simulink model "compressor"  (R2014a)
settings: Solver=ode45  StartTime=0.0  StopTime=100  RelTol=1e-4
libraries: simulink x2
settings Model: Creator=Max  LastModifiedBy=Max

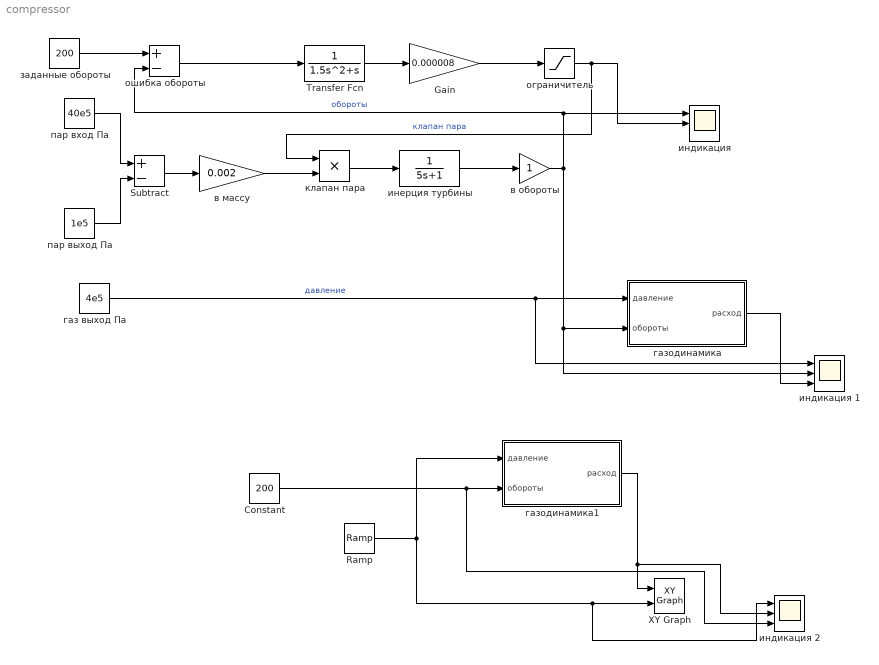
== system compressor ==
  Constant : Constant  Value=200
  Gain : Gain  Gain=0.000008
  Ramp : simulink/Sources/Ramp  slope=1  start=0  X0=1
  Subtract : Sum  Inputs=+-
  Transfer Fcn : TransferFcn  Denominator=[1.5 1 0]
  XY Graph : simulink/Sinks/XY Graph  xmin=-1500  xmax=1500  ymin=-50  ymax=50  st=-1
  в массу : Gain  Gain=0.002
  в обороты : Gain
  газ выход Па : Constant  Value=4e5
  газодинамика : Subsystem  TreatAsAtomicUnit=on
  газодинамика1 : Subsystem  TreatAsAtomicUnit=on
  заданные обороты : Constant  Value=200
  "индикация " : Scope  NumInputPorts=3
      settings: ShowLegends=on  YMin=0~-5~-5  YMax=4250~5~5
  индикация 1 : Scope  NumInputPorts=3
      settings: ShowLegends=on  YMin=-5~-5~-5  YMax=5~5~5
  индикация 2 : Scope  NumInputPorts=3
      settings: ShowLegends=on  YMin=-5~-5~-5  YMax=5~5~5  SaveName=ScopeData2
  инерция турбины : TransferFcn  Denominator=[5 1]
  клапан пара : Product
  ограничитель : Saturate  UpperLimit=1  LowerLimit=0
  ошибка обороты : Sum  Inputs=+-
  пар вход Па : Constant  Value=40e5
  пар выход Па : Constant  Value=1e5
  wires:
  пар выход Па/1 -> Subtract/2
  пар вход Па/1 -> Subtract/1
  Subtract/1 -> в массу/1
  в массу/1 -> клапан пара/2
  клапан пара/1 -> инерция турбины/1
  инерция турбины/1 -> в обороты/1
  заданные обороты/1 -> ошибка обороты/1
  в обороты/1 -> газодинамика/2(обороты), индикация 1/2, ошибка обороты/2, "индикация "/1  "обороты"
  ограничитель/1 -> клапан пара/1, "индикация "/2  "клапан пара"
  газ выход Па/1 -> газодинамика/1(давление), индикация 1/1  "давление"
  газодинамика/1(расход) -> индикация 1/3
  газодинамика1/1(расход) -> индикация 2/2, XY Graph/1
  Constant/1 -> индикация 2/3, газодинамика1/2(обороты)
  Ramp/1 -> индикация 2/1, XY Graph/2, газодинамика1/1(давление)
  Transfer Fcn/1 -> Gain/1
  ошибка обороты/1 -> Transfer Fcn/1
  Gain/1 -> ограничитель/1

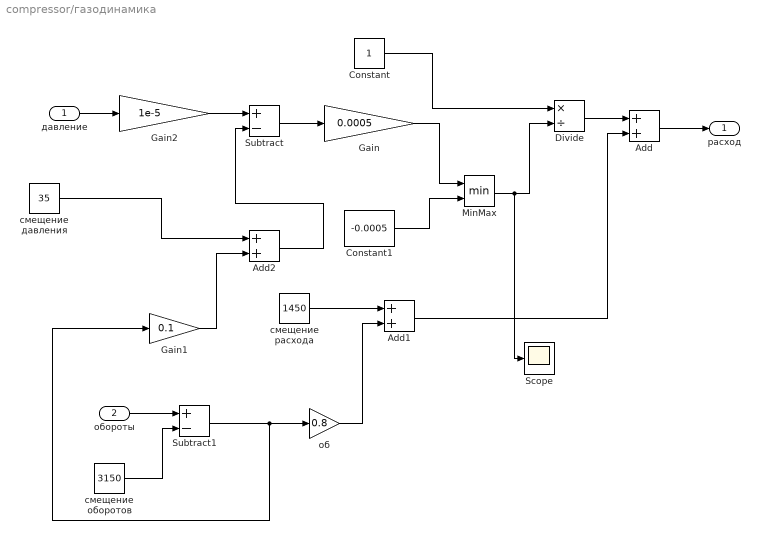
== system compressor/газодинамика ==
  давление : Inport
  обороты : Inport  Port=2
  Add : Sum
  Add1 : Sum
  Add2 : Sum
  Constant : Constant
  Constant1 : Constant  Value=-0.0005
  Divide : Product  Inputs=*/
  Gain : Gain  Gain=0.0005
  Gain1 : Gain  Gain=0.1
  Gain2 : Gain  Gain=1e-5
  MinMax : MinMax  Inputs=2
  Scope : Scope
      settings: SaveName=ScopeData4
  Subtract : Sum  Inputs=+-
  Subtract1 : Sum  Inputs=+-
  об : Gain  Gain=0.8
  смещение давления : Constant  Value=35
  смещение оборотов : Constant  Value=3150
  смещение расхода : Constant  Value=1450
  расход : Outport
  wires:
  смещение давления/1 -> Add2/1
  давление/1 -> Gain2/1
  Subtract/1 -> Gain/1
  смещение расхода/1 -> Add1/1
  Constant/1 -> Divide/1
  Divide/1 -> Add/1
  Add/1 -> расход/1
  обороты/1 -> Subtract1/1
  смещение оборотов/1 -> Subtract1/2
  Subtract1/1 -> Gain1/1, об/1
  Add1/1 -> Add/2
  об/1 -> Add1/2
  Gain1/1 -> Add2/2
  Add2/1 -> Subtract/2
  MinMax/1 -> Scope/1, Divide/2
  Gain/1 -> MinMax/1
  Constant1/1 -> MinMax/2
  Gain2/1 -> Subtract/1

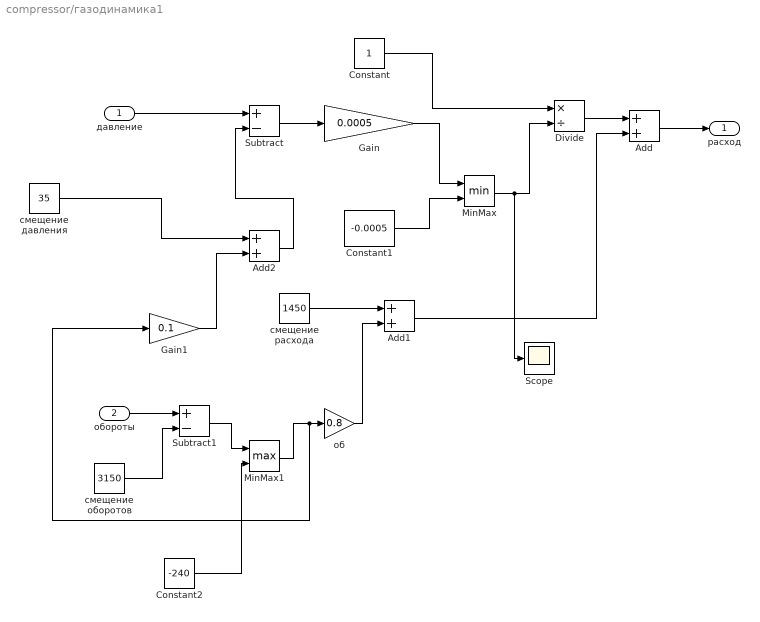
== system compressor/газодинамика1 ==
  давление : Inport
  обороты : Inport  Port=2
  Add : Sum
  Add1 : Sum
  Add2 : Sum
  Constant : Constant
  Constant1 : Constant  Value=-0.0005
  Constant2 : Constant  Value=-240
  Divide : Product  Inputs=*/
  Gain : Gain  Gain=0.0005
  Gain1 : Gain  Gain=0.1
  MinMax : MinMax  Inputs=2
  MinMax1 : MinMax  Function=max  Inputs=2
  Scope : Scope
      settings: SaveName=ScopeData3
  Subtract : Sum  Inputs=+-
  Subtract1 : Sum  Inputs=+-
  об : Gain  Gain=0.8
  смещение давления : Constant  Value=35
  смещение оборотов : Constant  Value=3150
  смещение расхода : Constant  Value=1450
  расход : Outport
  wires:
  смещение давления/1 -> Add2/1
  давление/1 -> Subtract/1
  Subtract/1 -> Gain/1
  смещение расхода/1 -> Add1/1
  Constant/1 -> Divide/1
  Divide/1 -> Add/1
  Add/1 -> расход/1
  обороты/1 -> Subtract1/1
  смещение оборотов/1 -> Subtract1/2
  MinMax1/1 -> Gain1/1, об/1
  об/1 -> Add1/2
  Gain1/1 -> Add2/2
  MinMax/1 -> Scope/1, Divide/2
  Gain/1 -> MinMax/1
  Constant1/1 -> MinMax/2
  Add2/1 -> Subtract/2
  Add1/1 -> Add/2
  Constant2/1 -> MinMax1/2
  Subtract1/1 -> MinMax1/1
